simulink model "test_biflat_unflat"  (R2019a)
settings: Solver=VariableStepAuto  StartTime=0.0  StopTime=10.0  RelTol=1e-3
libraries: ad_blocks x4
settings Model: Creator=eruffaldi  LastModifiedBy=eruffaldi

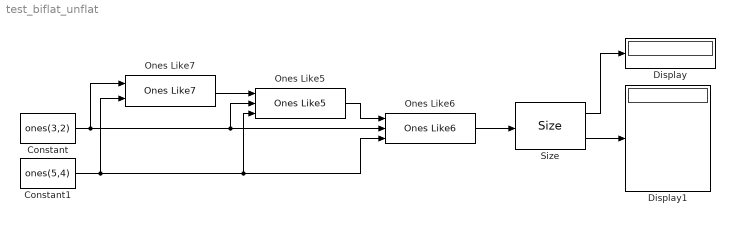
== system test_biflat_unflat ==
  Constant : Constant  Value=ones(3,2)
  Constant1 : Constant  Value=ones(5,4)
  Display : Display
  Display1 : Display
  Ones Like5 : ad_blocks/Ones Like5  SimulateUsing=Code generation
  Ones Like6 : ad_blocks/Ones Like6  SimulateUsing=Code generation
  Ones Like7 : ad_blocks/Ones Like7  SimulateUsing=Code generation
  Size : ad_blocks/Size  SystemSampleTime=-1
  wires:
  Constant/1 -> Ones Like5/2, Ones Like6/2, Ones Like7/1
  Constant1/1 -> Ones Like7/2, Ones Like5/3, Ones Like6/3
  Ones Like5/1 -> Ones Like6/1
  Ones Like6/1 -> Size/1
  Size/1 -> Display/1
  Ones Like7/1 -> Ones Like5/1
  Size/2 -> Display1/1
